simulink model "thingspeak_task"  (Simulink 3.00)
undefined symbols (not defined in the file): application, json
libraries: stringlib x4, mathlib x2, speclib x1, genlib x1

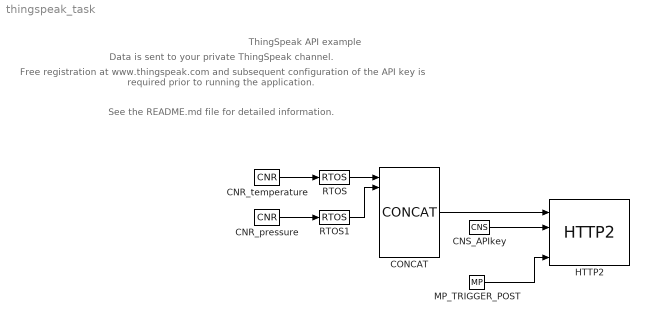
== system thingspeak_task ==
  note: ThingSpeak API example
  note: See the README.md file for detailed information.
  note: Free registration at www.thingspeak.com and subsequent configuration of
      | the API key is required prior to running the application.
  note: Data is sent to your private ThingSpeak channel.
  CNR_pressure : mathlib/CNR  ycn=105
  CNR_temperature : mathlib/CNR  ycn=9.81
  CNS_APIkey : stringlib/CNS  scv=YourThingSpeakAPIKey  nmax=0
  CONCAT : stringlib/CONCAT  ptrn="{ \"field1\": %1, \"field2\": %2 }"  nmax=0
  HTTP2 : speclib/HTTP2  url=https://api.thingspeak.com/update.json?api_key=  method=2: POST  VERIFY=off  postmime=application/json  acceptmime=application/json  timeout=5  BLOCKING=off  nmax=0  postmax=256  datamax=1024
  MP_TRIGGER_POST : genlib/MP  BSTATE=off  pwidth=1  RPTF=off
  RTOS : stringlib/RTOS  prec=3  mode=2: normal
  RTOS1 : stringlib/RTOS  prec=0  mode=2: normal
  wires:
  CNR_pressure/1 -> RTOS1/1
  CNR_temperature/1 -> RTOS/1
  CNS_APIkey/1 -> HTTP2/2
  CONCAT/1 -> HTTP2/1
  MP_TRIGGER_POST/1 -> HTTP2/4
  RTOS/1 -> CONCAT/1
  RTOS1/1 -> CONCAT/2
